simulink model "hand_linear_analyse"  (R2019b)
settings: Solver=ode4  StartTime=0.0  StopTime=20  FixedStep=0.001  RelTol=1e-3
undefined symbols (not defined in the file or in its folder): num, UAV
libraries: simulink_extras x14
settings Model: Creator=12572  LastModifiedBy=meiying
settings SolverCC: AlgebraicLoopSolver=LineSearch

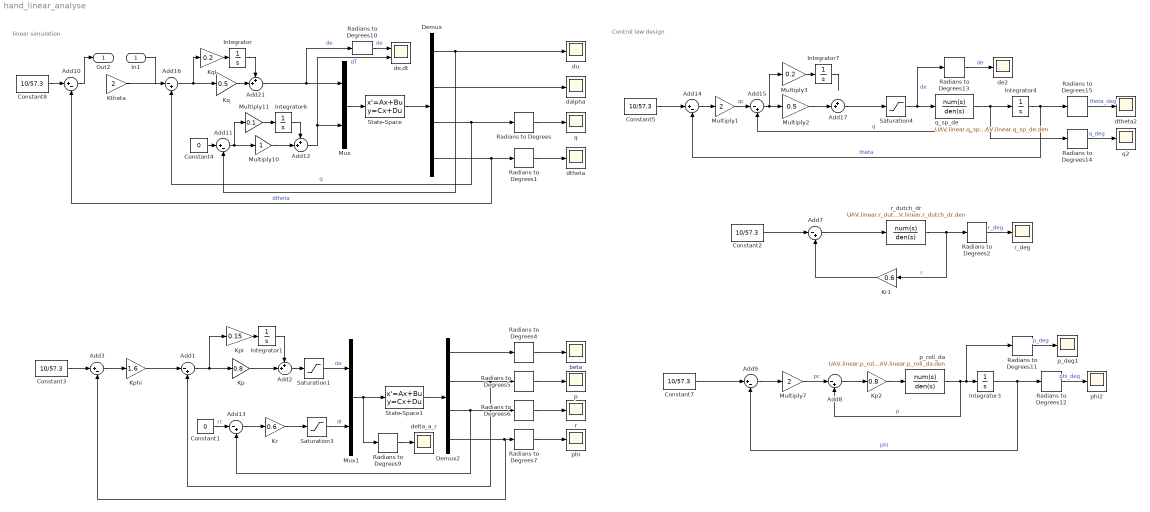
== system hand_linear_analyse ==
  note: Control law design
  note: linear simulation
  In1 : Inport
  Add{1,7..8,13,15..16} (6 alike) : Sum  Inputs=|-+
  Add{3,9..11,14} (5 alike) : Sum  Inputs=|+-
  Add{2,12,17,21} (4 alike) : Sum  Inputs=++|
  Constant1 : Constant  Value=0
  Constant{2..3,5,7..8} (5 alike) : Constant  Value=10/57.3
  Constant4 : Constant  Value=0
  Demux : Demux
  Demux2 : Demux
  Integrator{,1,3..4,6..7} (6 alike) : Integrator
  Kp : Gain  Gain=0.8
  Kp2 : Gain  Gain=0.8
  KpI : Gain  Gain=0.15
  Kphi : Gain  Gain=1.6
  Kq : Gain  Gain=0.5
  KqI : Gain  Gain=0.2
  Kr : Gain  Gain=0.6
  Kr1 : Gain  Gain=0.6
  Ktheta : Gain  Gain=2
  Multiply1 : Gain  Gain=2
  Multiply10 : Gain
  Multiply11 : Gain  Gain=0.1
  Multiply2 : Gain  Gain=0.5
  Multiply3 : Gain  Gain=0.2
  Multiply7 : Gain  Gain=2
  Mux : Mux  Inputs=2
  Mux1 : Mux  Inputs=2
  Radians to Degrees{,1..2,4..7,9..15} (14 alike) : simulink_extras/Transformations/Radians to Degrees
  Saturation1 : Saturate  UpperLimit=20/57.3  LowerLimit=-20/57.3
  Saturation3 : Saturate  UpperLimit=20/57.3  LowerLimit=-20/57.3
  Saturation4 : Saturate  UpperLimit=20/57.3  LowerLimit=-20/57.3
  State-Space : StateSpace  A=UAV.designpoint.longitudial.A(:,:,num)  B=UAV.designpoint.longitudial.B(:,:,num)  C=eye(4)  D=zeros(4,2)  InitialCondition=[0;0;0;0]
  State-Space1 : StateSpace  A=UAV.designpoint.lateral.A(:,:,num)  B=UAV.designpoint.lateral.B(:,:,num)  C=eye(4)  D=zeros(4,2)  InitialCondition=[0;0;0;0]
  beta : Scope
  dalpha : Scope
  de,dt : Scope  NumInputPorts=2
  de2 : Scope
  delta_a_r : Scope
  dtheta : Scope
  dtheta2 : Scope
  du : Scope
  p : Scope
  p_deg1 : Scope
  p_roll_da : TransferFcn  Numerator=UAV.linear.p_roll_da.num  Denominator=UAV.linear.p_roll_da.den
  phi : Scope
  phi2 : Scope
  q : Scope
  q2 : Scope
  q_sp_de : TransferFcn  Numerator=UAV.linear.q_sp_de.num  Denominator=UAV.linear.q_sp_de.den
  r : Scope
  r_deg : Scope
  r_dutch_dr : TransferFcn  Numerator=UAV.linear.r_dutch_dr.num  Denominator=UAV.linear.r_dutch_dr.den
  Out2 : Outport
  wires:
  Demux/4 -> Radians to Degrees1/1, Add10/2  "dtheta"
  Radians to Degrees1/1 -> dtheta/1
  Radians to Degrees/1 -> q/1
  Mux1/1 -> Radians to Degrees9/1, State-Space1/1
  State-Space/1 -> Demux/1
  Kq/1 -> Add21/2
  KqI/1 -> Integrator/1
  Add21/1 -> Radians to Degrees10/1, Mux/1  "de"
  Demux/2 -> dalpha/1
  Integrator/1 -> Add21/1
  Demux/3 -> Radians to Degrees/1, Add16/2  "q"
  Add16/1 -> KqI/1, Kq/1
  Add12/1 -> Mux/2, de,dt/2  "dT"
  Constant8/1 -> Add10/1
  Ktheta/1 -> ?
  Add10/1 -> Out2/1
  Demux/1 -> du/1, Add11/2
  Radians to Degrees6/1 -> r/1
  Radians to Degrees7/1 -> phi/1
  Radians to Degrees4/1 -> beta/1
  Demux2/3 -> Add13/2, Radians to Degrees6/1
  Demux2/2 -> Radians to Degrees5/1, Add1/2
  Demux2/1 -> Radians to Degrees4/1
  Radians to Degrees5/1 -> p/1
  State-Space1/1 -> Demux2/1
  Saturation1/1 -> Mux1/1  "da"
  Kphi/1 -> Add1/1
  Add1/1 -> Kp/1, KpI/1
  Integrator1/1 -> Add2/1
  KpI/1 -> Integrator1/1
  Kp/1 -> Add2/2
  Constant3/1 -> Add3/1
  Add3/1 -> Kphi/1
  Demux2/4 -> Add3/2, Radians to Degrees7/1
  Mux/1 -> State-Space/1
  Saturation3/1 -> Mux1/2  "dr"
  Radians to Degrees9/1 -> delta_a_r/1
  Radians to Degrees10/1 -> de,dt/1  "de"
  Add2/1 -> Saturation1/1
  Constant4/1 -> Add11/1
  Add11/1 -> Multiply11/1, Multiply10/1
  Integrator6/1 -> Add12/1
  Multiply11/1 -> Integrator6/1
  Multiply10/1 -> Add12/2
  Add13/1 -> Kr/1
  Integrator4/1 -> Radians to Degrees15/1, Add14/2  "theta"
  Radians to Degrees14/1 -> q2/1  "q_deg"
  Radians to Degrees13/1 -> de2/1  "de"
  Add14/1 -> Multiply1/1
  Radians to Degrees15/1 -> dtheta2/1  "theta_deg"
  Multiply3/1 -> Integrator7/1
  Integrator7/1 -> ?
  Constant5/1 -> Add14/1
  Saturation4/1 -> q_sp_de/1, Radians to Degrees13/1  "de"
  q_sp_de/1 -> Integrator4/1, Add15/2, Radians to Degrees14/1  "q"
  Add15/1 -> Multiply2/1, Multiply3/1
  Multiply2/1 -> Add17/2
  Multiply1/1 -> Add15/1  "qc"
  Radians to Degrees2/1 -> r_deg/1  "r_deg"
  r_dutch_dr/1 -> Kr1/1, Radians to Degrees2/1  "r"
  Constant2/1 -> Add7/1
  Add7/1 -> r_dutch_dr/1
  Kr1/1 -> Add7/2
  Radians to Degrees11/1 -> p_deg1/1  "p_deg"
  p_roll_da/1 -> Radians to Degrees11/1, Integrator3/1, Add8/2  "p"
  Add8/1 -> Kp2/1
  Add9/1 -> Multiply7/1
  Radians to Degrees12/1 -> phi2/1  "phi_deg"
  Integrator3/1 -> Radians to Degrees12/1, Add9/2  "phi"
  Multiply7/1 -> Add8/1  "pc"
  Constant7/1 -> Add9/1
  Kp2/1 -> p_roll_da/1
  Add17/1 -> Saturation4/1
  Constant1/1 -> Add13/1  "rc"
  Kr/1 -> Saturation3/1
  In1/1 -> Add16/1
